simulink model "Ej5_v2"  (R2015a)
settings: Solver=ode45  StartTime=0.0  StopTime=10.0  RelTol=1e-3
libraries: cstblocks x4, simulink x2
settings Model: Creator=Daniel  LastModifiedBy=Daniel

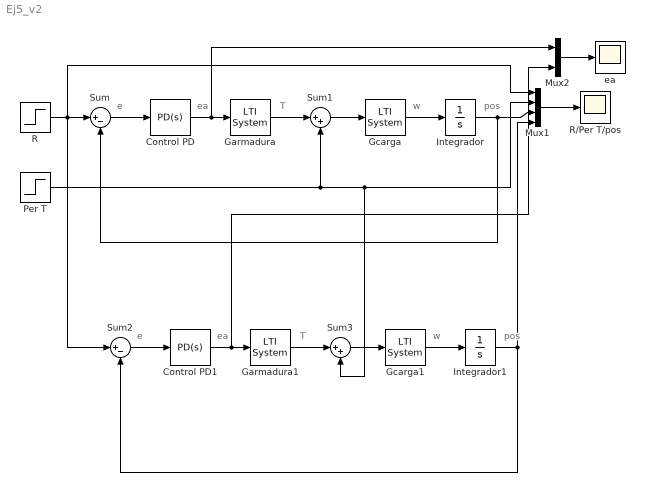
== system Ej5_v2 ==
  note: T
  note: pos
  note: w
  note: e
  note: ea
  note: T
  note: pos
  note: w
  note: e
  note: ea
  Control PD : simulink/Continuous/PID Controller  Controller=PD  TimeDomain=Continuous-time  SampleTime=-1  IntegratorMethod=Forward Euler  FilterMethod=Forward Euler  Form=Ideal  UseFilter=on  ControllerParametersSource=internal  P=120  I=0  D=0.05  N=2000  InitialConditionSource=internal  InitialConditionForIntegrator=0  InitialConditionForFilter=0  ExternalReset=none  LimitOutput=off  UpperSaturationLimit=12  LowerSaturationLimit=-inf  LinearizeAsGain=on  AntiWindupMode=none  Kb=1  TrackingMode=off  Kt=1  PParamMin=[]  PParamMax=[]  IParamMin=[]  IParamMax=[]  DParamMin=[]  DParamMax=[]  NParamMin=[]  NParamMax=[]  KbParamMin=[]  KbParamMax=[]  KtParamMin=[]  KtParamMax=[]  POutMin=[]  POutMax=[]  IOutMin=[]  IOutMax=[]  DOutMin=[]  DOutMax=[]  NOutMin=[]  NOutMax=[]  KbOutMin=[]  KbOutMax=[]  KtOutMin=[]  KtOutMax=[]  IntegratorOutMin=[]  IntegratorOutMax=[]  FilterOutMin=[]  FilterOutMax=[]  SumOutMin=[]  SumOutMax=[]  SumI1OutMin=[]  SumI1OutMax=[]  SumI2OutMin=[]  SumI2OutMax=[]  SumI3OutMin=[]  SumI3OutMax=[]  SumDOutMin=[]  SumDOutMax=[]  SaturationOutMin=[]  SaturationOutMax=[]  IntegratorContinuousStateAttributes=''  IntegratorStateMustResolveToSignalObject=off  IntegratorRTWStateStorageClass=Auto  FilterContinuousStateAttributes=''  FilterStateMustResolveToSignalObject=off  FilterRTWStateStorageClass=Auto  DifferentiatorICPrevScaledInput=0  DifferentiatorOutMin=[]  DifferentiatorOutMax=[]
  Control PD1 : simulink/Continuous/PID Controller  Controller=PD  TimeDomain=Continuous-time  SampleTime=-1  IntegratorMethod=Forward Euler  FilterMethod=Forward Euler  Form=Ideal  UseFilter=on  ControllerParametersSource=internal  P=120  I=0  D=0.05  N=2000  InitialConditionSource=internal  InitialConditionForIntegrator=0  InitialConditionForFilter=0  ExternalReset=none  LimitOutput=on  UpperSaturationLimit=12  LowerSaturationLimit=-inf  LinearizeAsGain=on  AntiWindupMode=none  Kb=1  TrackingMode=off  Kt=1  PParamMin=[]  PParamMax=[]  IParamMin=[]  IParamMax=[]  DParamMin=[]  DParamMax=[]  NParamMin=[]  NParamMax=[]  KbParamMin=[]  KbParamMax=[]  KtParamMin=[]  KtParamMax=[]  POutMin=[]  POutMax=[]  IOutMin=[]  IOutMax=[]  DOutMin=[]  DOutMax=[]  NOutMin=[]  NOutMax=[]  KbOutMin=[]  KbOutMax=[]  KtOutMin=[]  KtOutMax=[]  IntegratorOutMin=[]  IntegratorOutMax=[]  FilterOutMin=[]  FilterOutMax=[]  SumOutMin=[]  SumOutMax=[]  SumI1OutMin=[]  SumI1OutMax=[]  SumI2OutMin=[]  SumI2OutMax=[]  SumI3OutMin=[]  SumI3OutMax=[]  SumDOutMin=[]  SumDOutMax=[]  SaturationOutMin=[]  SaturationOutMax=[]  IntegratorContinuousStateAttributes=''  IntegratorStateMustResolveToSignalObject=off  IntegratorRTWStateStorageClass=Auto  FilterContinuousStateAttributes=''  FilterStateMustResolveToSignalObject=off  FilterRTWStateStorageClass=Auto  DifferentiatorICPrevScaledInput=0  DifferentiatorOutMin=[]  DifferentiatorOutMax=[]
  Garmadura : cstblocks/LTI System  sys=Garm  IC=[]
  Garmadura1 : cstblocks/LTI System  sys=Garm  IC=[]
  Gcarga : cstblocks/LTI System  sys=Gcar  IC=[]
  Gcarga1 : cstblocks/LTI System  sys=Gcar  IC=[]
  Integrador : Integrator
  Integrador1 : Integrator
  Mux1 : Mux
  Mux2 : Mux  Inputs=2
  Per T : Step  SampleTime=0
  R : Step  Time=0  After=0.6  SampleTime=0
  R/Per T/pos : Scope
      settings: SaveName=pos
  Sum : Sum  Inputs=|+-
  Sum1 : Sum  Inputs=|++
  Sum2 : Sum  Inputs=|+-
  Sum3 : Sum  Inputs=|++
  "ea " : Scope
      settings: SaveName=ea
  wires:
  Sum/1 -> Control PD/1
  Control PD/1 -> Mux2/1, Garmadura/1
  Gcarga/1 -> Integrador/1
  Mux1/1 -> R/Per T/pos/1
  Integrador/1 -> Mux1/3, Sum/2
  Garmadura/1 -> Sum1/1
  Sum1/1 -> Gcarga/1
  Per T/1 -> Sum1/2, Sum3/2, Mux1/2
  Mux2/1 -> "ea "/1
  Sum2/1 -> Control PD1/1
  Control PD1/1 -> Mux2/2, Garmadura1/1
  Gcarga1/1 -> Integrador1/1
  R/1 -> Sum2/1, Mux1/1, Sum/1
  Integrador1/1 -> Mux1/4, Sum2/2
  Garmadura1/1 -> Sum3/1
  Sum3/1 -> Gcarga1/1
